simulink model "ModelRed"  (R2024b)
settings: Solver=VariableStepAuto  StartTime=0.0  StopTime=10.0  RelTol=1e-3
settings Model: Creator=Dr.Red  LastModifiedBy=Dr.Red
settings DataIOCC: ReturnWorkspaceOutputs=off
settings ModelReferenceCC: PropagateSignalLabelsOutOfModel=off

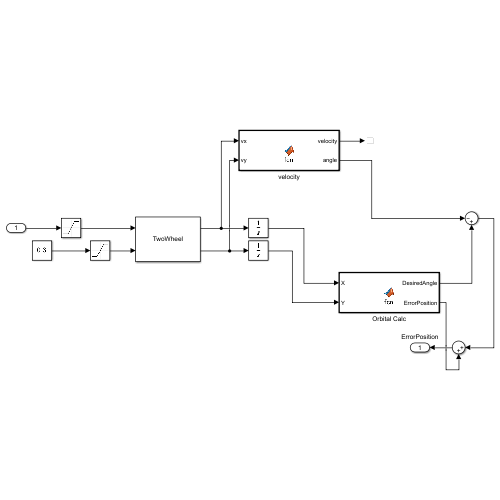
[thumbnail: Simulink's stored preview of the top-level diagram]
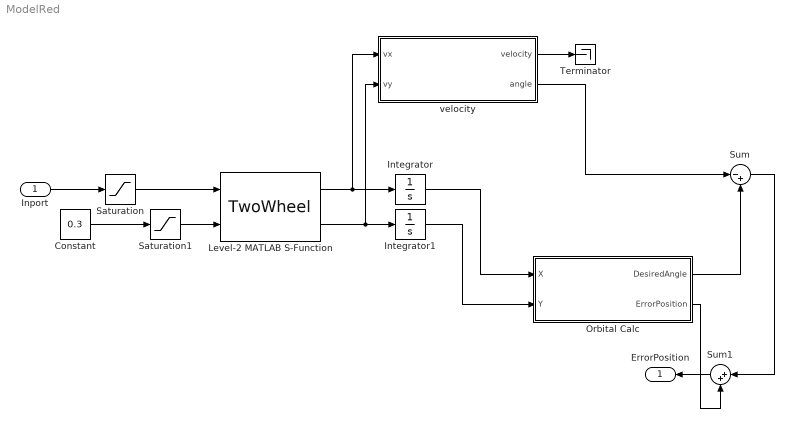
== system ModelRed ==
  Inport : Inport
  Constant : Constant  Value=0.3
  Integrator : Integrator
  Integrator1 : Integrator
  Level-2 MATLAB S-Function : M-S-Function  FunctionName=TwoWheel  Parameters=10,0,0,0
  Orbital Calc : MATLAB Function  TreatAsAtomicUnit=on
  Saturation : Saturate  UpperLimit=0.3  LowerLimit=-0.3
  Saturation1 : Saturate  UpperLimit=1.5  LowerLimit=-2
  Sum : Sum  Inputs=|-+
  Sum1 : Sum  Inputs=|++
  Terminator : Terminator
  velocity : MATLAB Function  TreatAsAtomicUnit=on
  ErrorPosition : Outport
  wires:
  velocity/2(angle) -> Sum/1
  Orbital Calc/1(DesiredAngle) -> Sum/2
  Inport/1 -> Saturation/1
  Level-2 MATLAB S-Function/2 -> velocity/2(vy), Integrator1/1
  Saturation1/1 -> Level-2 MATLAB S-Function/2
  Saturation/1 -> Level-2 MATLAB S-Function/1
  Integrator1/1 -> Orbital Calc/2(Y)
  Integrator/1 -> Orbital Calc/1(X)
  Level-2 MATLAB S-Function/1 -> velocity/1(vx), Integrator/1
  Constant/1 -> Saturation1/1
  velocity/1(velocity) -> Terminator/1
  Sum/1 -> Sum1/1
  Sum1/1 -> ErrorPosition/1
  Orbital Calc/2(ErrorPosition) -> Sum1/2

== matlab function ModelRed/Orbital Calc ==
  data: DesiredAngle output; X input; ErrorPosition output; Y input
function [DesiredAngle,ErrorPosition] = fcn(X,Y)
    
    RoundPosition = [0,15];

    Radius = 15;

ErrorPosition = - Radius + power((RoundPosition(1)-X)^2+(RoundPosition(2)-Y)^2,0.5);

DesiredAngle = atan2(X-RoundPosition(1),RoundPosition(2)-Y);

== matlab function ModelRed/velocity ==
  data: vx input; velocity output; vy input; angle output
function [velocity,angle] = fcn(vx,vy)
    

velocity = power(vx^2+vy^2,0.5);

angle = atan2(vy,vx);
